simulink model "EPC9118_Buck"  (R2019b)
settings: Solver=VariableStepAuto  StartTime=0.0  StopTime=5000/fs  MaxStep=2.5e-8  RelTol=1e-3
values from neighbouring files (symbols this model uses):
  fs = 400e3    (= 400000)    [Buck_simulink.m]
undefined symbols (not defined in the file or in its folder): plecs
libraries: powerlib_meascontrol x4
settings Model: Creator=jb  LastModifiedBy=jb

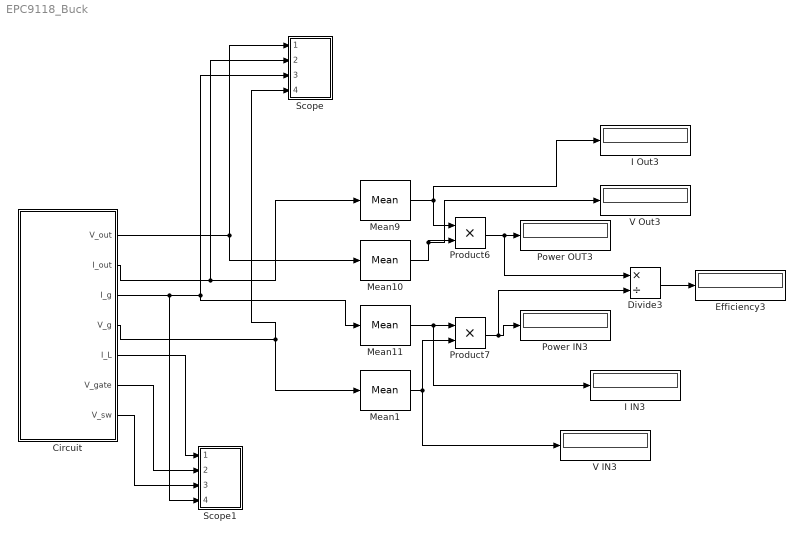
== system EPC9118_Buck ==
  Circuit : Subsystem  LoadFcn=plecs('sl', 200);  InitFcn=plecs('sl', 214);  StartFcn=plecs('sl', 208);  StopFcn=plecs('sl', 209);  mask(PlecsCircuit){PLECSData=<binary blob, 2972 chars, not shown>}
      mask prompts: PLECSData "PLECS Data (Do not delete or modify!)"
      mask init:
      | % PLACE CUSTOM INITIALIZATIONS ABOVE
      | % DO NOT REMOVE
      | plecs('sl', 215);
      | % DO NOT REMOVE
      settings: CopyFcn=plecs('sl', 203);  DeleteFcn=plecs('sl', 205);  UndoDeleteFcn=plecs('sl', 206);  PreSaveFcn=plecs('sl', 211);  PostSaveFcn=plecs('sl', 201);  NameChangeFcn=plecs('sl', 210);  DestroyFcn=plecs('sl', 207);  PreCopyFcn=plecs('sl', 216);  OpenFcn=plecs('sl', 202);  ErrorFcn=plerrorfcn
      mask Help: web(['file:///' fullfile(plecsdoc, 'creatingacircuit.html')])
      mask Display: disp('PLECS\nCircuit')
  Divide3 : Product  Inputs=*/
  Efficiency3 : Display
  I IN3 : Display
  I Out3 : Display
  Mean{1,9..11} (4 alike) : powerlib_meascontrol/Measurements/Mean  Freq=fs/10  Vinit=0  Ts=0
      settings: SourceProductName=Simscape Electrical
  Power IN3 : Display
  Power OUT3 : Display
  Product6 : Product
  Product7 : Product
  Scope : Subsystem  LoadFcn=plecs('sl', 300);  InitFcn=plecs('sl', 314);  StartFcn=plecs('sl', 308);  StopFcn=plecs('sl', 309);  mask{Settings=<binary blob, 1468 chars, not shown>}
      mask init:
      | plecs('sl', 315);
      settings: CopyFcn=plecs('sl', 303);  DeleteFcn=plecs('sl', 305);  UndoDeleteFcn=plecs('sl', 306);  PreSaveFcn=plecs('sl', 311);  NameChangeFcn=plecs('sl', 310);  DestroyFcn=plecs('sl', 307);  OpenFcn=plecs('sl', 302);  ErrorFcn=plerrorfcn
      mask Display: plot([0.1 0.9 0.9 0.1 0.1], [0.9 0.9 0.5 0.5 0.9])
  Scope1 : Subsystem  LoadFcn=plecs('sl', 300);  InitFcn=plecs('sl', 314);  StartFcn=plecs('sl', 308);  StopFcn=plecs('sl', 309);  mask{Settings=<binary blob, 1468 chars, not shown>}
      mask init:
      | plecs('sl', 315);
      settings: CopyFcn=plecs('sl', 303);  DeleteFcn=plecs('sl', 305);  UndoDeleteFcn=plecs('sl', 306);  PreSaveFcn=plecs('sl', 311);  NameChangeFcn=plecs('sl', 310);  DestroyFcn=plecs('sl', 307);  OpenFcn=plecs('sl', 302);  ErrorFcn=plerrorfcn
      mask Display: plot([0.1 0.9 0.9 0.1 0.1], [0.9 0.9 0.5 0.5 0.9])
  V IN3 : Display
  V Out3 : Display
  wires:
  Mean11/1 -> I IN3/1, Product7/1
  Divide3/1 -> Efficiency3/1
  Mean1/1 -> V IN3/1, Product7/2
  Mean9/1 -> Product6/1, I Out3/1
  Product7/1 -> Divide3/2, Power IN3/1
  Product6/1 -> Divide3/1, Power OUT3/1
  Mean10/1 -> V Out3/1, Product6/2
  Circuit/4(V_g) -> Mean1/1, Scope/4(4)
  Circuit/3(I_g) -> Scope1/4(4), Mean11/1, Scope/3(3)
  Circuit/2(I_out) -> Scope/2(2), Mean9/1
  Circuit/1(V_out) -> Scope/1(1), Mean10/1
  Circuit/5(I_L) -> Scope1/1(1)
  Circuit/6(V_gate) -> Scope1/2(2)
  Circuit/7(V_sw) -> Scope1/3(3)

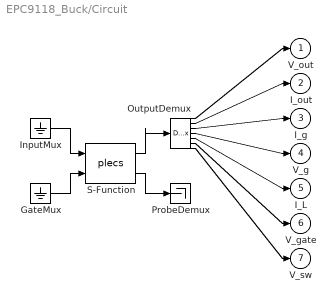
== system EPC9118_Buck/Circuit ==
  " GateMux " : Ground
  " InputMux " : Ground
  " OutputDemux " : Demux  Outputs=[ 1 1 1 1 1 2 1 ]
  " ProbeDemux " : Terminator
  " S-Function " : S-Function  FunctionName=plecs  SFunctionDeploymentMode=off  EnableBusSupport=off
  V_out : Outport  PortDimensions=1
  I_out : Outport  Port=2  PortDimensions=1
  I_g : Outport  Port=3  PortDimensions=1
  V_g : Outport  Port=4  PortDimensions=1
  I_L : Outport  Port=5  PortDimensions=1
  V_gate : Outport  Port=6  PortDimensions=2
  V_sw : Outport  Port=7  PortDimensions=1
  wires:
  " S-Function "/1 -> " OutputDemux "/1
  " InputMux "/1 -> " S-Function "/1
  " GateMux "/1 -> " S-Function "/2
  " S-Function "/2 -> " ProbeDemux "/1
  " OutputDemux "/1 -> V_out/1
  " OutputDemux "/2 -> I_out/1
  " OutputDemux "/3 -> I_g/1
  " OutputDemux "/4 -> V_g/1
  " OutputDemux "/5 -> I_L/1
  " OutputDemux "/6 -> V_gate/1
  " OutputDemux "/7 -> V_sw/1

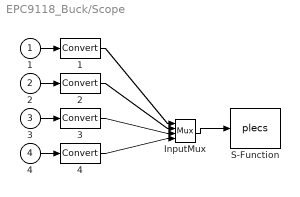
== system EPC9118_Buck/Scope ==
  1 : Inport
  2 : Inport  Port=2
  3 : Inport  Port=3
  4 : Inport  Port=4
  " 1 " : DataTypeConversion  SaturateOnIntegerOverflow=on  RndMeth=Zero
  " 2 " : DataTypeConversion  SaturateOnIntegerOverflow=on  RndMeth=Zero
  " 3 " : DataTypeConversion  SaturateOnIntegerOverflow=on  RndMeth=Zero
  " 4 " : DataTypeConversion  SaturateOnIntegerOverflow=on  RndMeth=Zero
  " InputMux " : Mux
  " S-Function " : S-Function  FunctionName=plecs  SFunctionDeploymentMode=off  EnableBusSupport=off
  wires:
  " InputMux "/1 -> " S-Function "/1
  1/1 -> " 1 "/1
  " 1 "/1 -> " InputMux "/1
  2/1 -> " 2 "/1
  " 2 "/1 -> " InputMux "/2
  3/1 -> " 3 "/1
  " 3 "/1 -> " InputMux "/3
  4/1 -> " 4 "/1
  " 4 "/1 -> " InputMux "/4

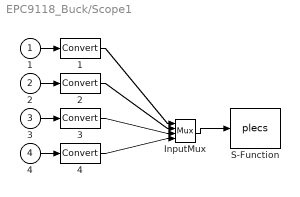
== system EPC9118_Buck/Scope1 ==
  1 : Inport
  2 : Inport  Port=2
  3 : Inport  Port=3
  4 : Inport  Port=4
  " 1 " : DataTypeConversion  SaturateOnIntegerOverflow=on  RndMeth=Zero
  " 2 " : DataTypeConversion  SaturateOnIntegerOverflow=on  RndMeth=Zero
  " 3 " : DataTypeConversion  SaturateOnIntegerOverflow=on  RndMeth=Zero
  " 4 " : DataTypeConversion  SaturateOnIntegerOverflow=on  RndMeth=Zero
  " InputMux " : Mux
  " S-Function " : S-Function  FunctionName=plecs  SFunctionDeploymentMode=off  EnableBusSupport=off
  wires:
  " InputMux "/1 -> " S-Function "/1
  1/1 -> " 1 "/1
  " 1 "/1 -> " InputMux "/1
  2/1 -> " 2 "/1
  " 2 "/1 -> " InputMux "/2
  3/1 -> " 3 "/1
  " 3 "/1 -> " InputMux "/3
  4/1 -> " 4 "/1
  " 4 "/1 -> " InputMux "/4
